simulink model "alba9_closed_loop"  (R2025a)
settings: Solver=ode15s  StartTime=0.0  StopTime=120  MaxStep=0.025  RelTol=2e-8  AbsTol=1e-7
values from neighbouring files (symbols this model uses):
  V0mL = P.V0*1e6    [alba9_check_ode.m]
undefined symbols (not defined in the file or in its folder): S_vec
settings Model: Creator=15886  LastModifiedBy=15886
settings DataIOCC: SaveOutput=off  SignalLogging=off  SaveTime=off

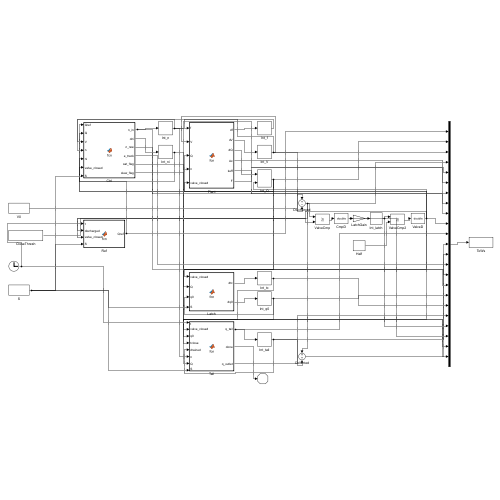
[thumbnail: Simulink's stored preview of the top-level diagram]
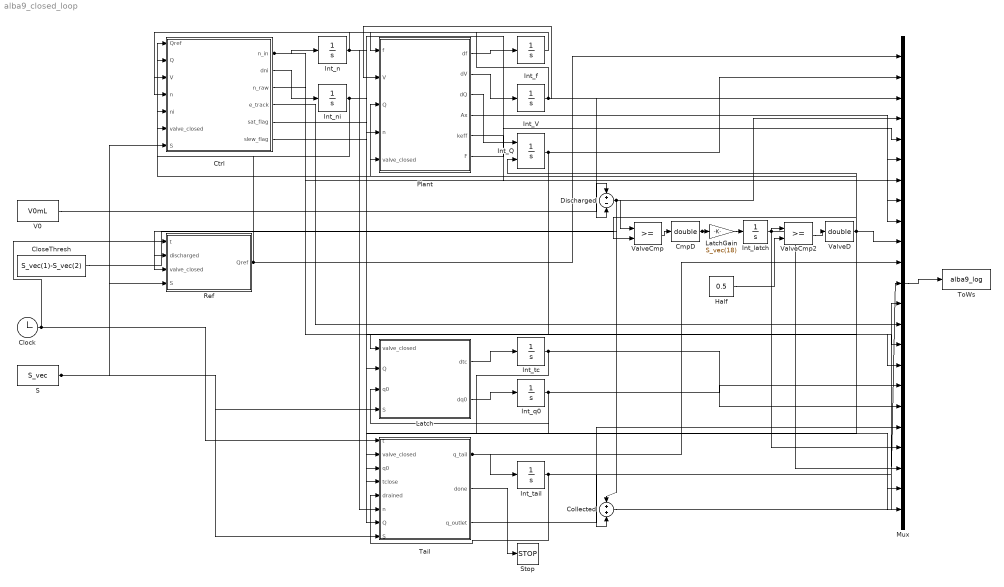
== system alba9_closed_loop ==
  Clock : Clock
  CloseThresh : Constant  Value=S_vec(1)-S_vec(2)
  CmpD : DataTypeConversion  OutDataTypeStr=double  SaturateOnIntegerOverflow=off  RndMeth=Floor
  Collected : Sum
  Ctrl : MATLAB Function  TreatAsAtomicUnit=on
  Discharged : Sum  Inputs=+-
  Half : Constant  Value=0.5
  Int_Q : Integrator  ExternalReset=rising  AbsoluteTolerance=1e-7
  Int_V : Integrator  InitialCondition=V0mL  AbsoluteTolerance=1e-7
  Int_f : Integrator  LimitOutput=on  LowerSaturationLimit=0  AbsoluteTolerance=1e-9
  Int_latch : Integrator  LimitOutput=on  UpperSaturationLimit=1  LowerSaturationLimit=0  AbsoluteTolerance=1e-9
  Int_n : Integrator  LimitOutput=on  UpperSaturationLimit=S_vec(12)  LowerSaturationLimit=0  AbsoluteTolerance=1e-4
  Int_ni : Integrator  AbsoluteTolerance=1e-4
  Int_q0 : Integrator  AbsoluteTolerance=1e-7
  Int_tail : Integrator  AbsoluteTolerance=1e-9
  Int_tc : Integrator  AbsoluteTolerance=1e-7
  Latch : MATLAB Function  TreatAsAtomicUnit=on
  LatchGain : Gain  Gain=S_vec(18)
  Mux : Mux  Inputs=23
  Plant : MATLAB Function  TreatAsAtomicUnit=on
  Ref : MATLAB Function  TreatAsAtomicUnit=on
  S : Constant  Value=S_vec
  Stop : Stop
  Tail : MATLAB Function  TreatAsAtomicUnit=on
  ToWs : ToWorkspace  VariableName=alba9_log  SaveFormat=Structure With Time  SampleTime=-1
  V0 : Constant  Value=V0mL
  ValveCmp : RelationalOperator  OutDataTypeStr=boolean  RndMeth=Simplest  InputSameDT=off
  ValveCmp2 : RelationalOperator  OutDataTypeStr=boolean  RndMeth=Simplest  InputSameDT=off
  ValveD : DataTypeConversion  OutDataTypeStr=double  SaturateOnIntegerOverflow=off  RndMeth=Floor
  wires:
  Int_f/1 -> Plant/1(f)
  Int_V/1 -> Plant/2(V), Discharged/2, Ctrl/3(V), Mux/3
  Int_Q/1 -> Plant/3(Q), Ctrl/2(Q), Latch/2(Q), Tail/7(Q), Mux/2
  Int_n/1 -> Plant/4(n), Ctrl/4(n), Tail/6(n), Mux/6
  ValveD/1 -> Plant/5(valve_closed), Int_Q/2, Ref/3(valve_closed), Ctrl/6(valve_closed), Latch/1(valve_closed), Tail/2(valve_closed), Mux/10
  Plant/1(df) -> Int_f/1
  Plant/2(dV) -> Int_V/1
  Plant/3(dQ) -> Int_Q/1
  V0/1 -> Discharged/1
  Discharged/1 -> ValveCmp/1, Ref/2(discharged), Collected/1, Mux/4
  CloseThresh/1 -> ValveCmp/2
  ValveCmp/1 -> CmpD/1
  CmpD/1 -> LatchGain/1, Mux/21
  LatchGain/1 -> Int_latch/1
  Int_latch/1 -> ValveCmp2/1, Mux/20
  Half/1 -> ValveCmp2/2
  ValveCmp2/1 -> ValveD/1
  Clock/1 -> Ref/1(t), Tail/1(t)
  S/1 -> Ref/4(S), Ctrl/7(S), Latch/4(S), Tail/8(S)
  Ref/1(Qref) -> Ctrl/1(Qref), Mux/1
  Int_ni/1 -> Ctrl/5(ni), Mux/16
  Ctrl/1(n_in) -> Int_n/1, Mux/15
  Ctrl/2(dni) -> Int_ni/1
  Int_q0/1 -> Latch/3(q0), Tail/3(q0), Mux/17
  Latch/1(dtc) -> Int_tc/1
  Latch/2(dq0) -> Int_q0/1
  Int_tc/1 -> Tail/4(tclose), Mux/18
  Int_tail/1 -> Tail/5(drained), Collected/2, Mux/12
  Tail/1(q_tail) -> Int_tail/1, Mux/11
  Tail/2(done) -> Stop/1
  Plant/6(F) -> Mux/5
  Ctrl/3(n_raw) -> Mux/7
  Plant/5(keff) -> Mux/8
  Plant/4(Ax) -> Mux/9
  Collected/1 -> Mux/13
  Ctrl/4(e_track) -> Mux/14
  Tail/3(q_outlet) -> Mux/19
  Ctrl/5(sat_flag) -> Mux/22
  Ctrl/6(slew_flag) -> Mux/23
  Mux/1 -> ToWs/1

== matlab function alba9_closed_loop/Ctrl ==
  data: Qref input; n_in output; Q input; V input; n input; ni input; valve_closed input; S input; dni output; n_raw output; e_track output; sat_flag output; slew_flag output
function [n_in,dni,n_raw,e_track,sat_flag,slew_flag] = fcn(Qref,Q,V,n,ni,valve_closed,S)
%#codegen
[n_in,dni,n_raw,e_track,~,sat_flag,slew_flag] = ...
    alba9_controller(Qref,Q,V,n,ni,valve_closed,S);

== matlab function alba9_closed_loop/Ref ==
  data: t input; Qref output; discharged input; valve_closed input; S input
function Qref = fcn(t,discharged,valve_closed,S)
%#codegen
Qref = alba9_reference(t,discharged,valve_closed,S);

== matlab function alba9_closed_loop/Plant ==
  data: f input; df output; V input; Q input; n input; valve_closed input; dV output; dQ output; Ax output; keff output; F output
function [df,dV,dQ,Ax,keff,F] = fcn(f,V,Q,n,valve_closed)
%#codegen
P = alba9_const();
% false: Int_f is a saturated integrator, it enforces f >= 0 itself
[df,dV,dQ,Ax,keff,F] = alba9_plant(f,V,Q,n,valve_closed,P,false);

== matlab function alba9_closed_loop/Latch ==
  data: valve_closed input; dtc output; Q input; q0 input; S input; dq0 output
function [dtc,dq0] = fcn(valve_closed,Q,q0,S)
%#codegen
% Both integrators simply stop when the valve latches closed: Int_tc then
% holds the closing time and Int_q0 holds the flow it was tracking. Because
% the valve flag is monotone, they freeze exactly once and never restart.
% Int_q0 is a first-order tracker with time constant S(19), so the captured
% q0 is a LAGGED pre-closure flow, not the exact left limit of Q.
isopen = 1 - min(max(valve_closed,0),1);
dtc = isopen;
dq0 = isopen*(Q-q0)/S(19);

== matlab function alba9_closed_loop/Tail ==
  data: t input; q_tail output; valve_closed input; q0 input; tclose input; drained input; n input; Q input; S input; done output; q_outlet output
function [q_tail,done,q_outlet] = fcn(t,valve_closed,q0,tclose,drained,n,Q,S)
%#codegen
[q_tail,done,q_outlet] = alba9_tail(t,valve_closed,q0,tclose,drained,n,Q,S);
